simulink model "MODEL_PV"  (R2024a)
settings: Solver=VariableStepAuto  StartTime=0.0  StopTime=120  RelTol=1e-3
PostLoadFcn:
  | setup_01
model workspace (MAT data in the model file):
  TrafficLightPosition = [-6.9 -1.9 8]
  egoVelocity = 9
  relDist = inf
  relVelMIO = inf
  timeGap = 0.9
  trafficLightSensorStates = 1
undefined symbols (not defined in the file): costmap, intersectionInfo, maxMIOLeadDistance, posSelector, referencePathInfo, routePlan, sceneOrigin, Ts, v_set, velSelector
libraries: drivingscenarioandsensors x2, drivingvehiclecontroller x1
CloseFcn:
  | clearvars -except out
settings Model: PacingRate=0.500000  Creator=fidel  LastModifiedBy=L03509110
settings OptimizationCC: ReuseModelBlockBuffer=off
settings RTWCC: GPUComputeCapability=3.5

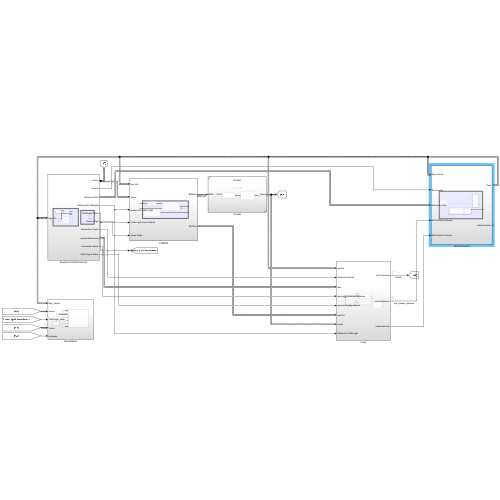
[thumbnail: Simulink's stored preview of the top-level diagram]
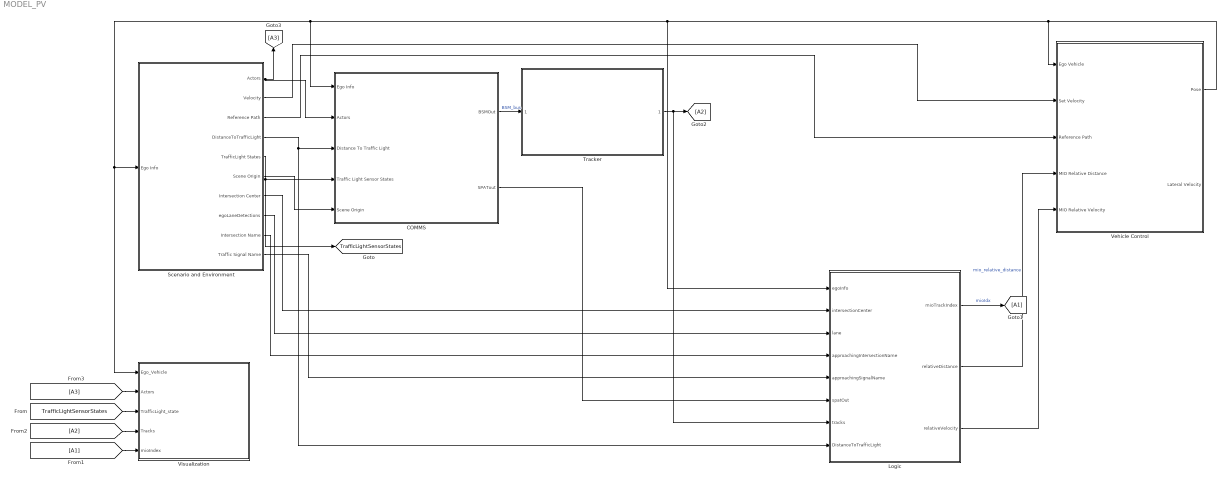
== system MODEL_PV ==
  COMMS : Subsystem
  Logic : Subsystem
  Scenario and Environment : Subsystem
  Tracker : Subsystem  ReferencedSubsystem=Tracker
  Vehicle Control : Subsystem
  Visualization : Subsystem
  tag scope: TrafficLightSensorStates=global
  wires:
  Vehicle Control/1(Pose) -> Vehicle Control/1(Ego Vehicle), Logic/1(egoInfo), COMMS/1(Ego Info), Visualization/1(Ego_Vehicle), Scenario and Environment/1(Ego Info)
  Scenario and Environment/3(Reference Path) -> Vehicle Control/3(Reference Path)
  [A3] -> Visualization/2(Actors)
  Scenario and Environment/1(Actors) -> [A3], COMMS/2(Actors)
  [TrafficLightSensorStates] -> Visualization/3(TrafficLight_state)
  [A2] -> Visualization/4(Tracks)
  [A1] -> Visualization/5(mioIndex)
  Scenario and Environment/2(Velocity) -> Vehicle Control/2(Set Velocity)
  Scenario and Environment/4(DistanceToTrafficLight) -> Logic/8(DistanceToTrafficLight), COMMS/3("Distance To Traffic Light ")
  Scenario and Environment/5(TrafficLight States) -> [TrafficLightSensorStates], COMMS/4(Traffic Light Sensor States)
  Scenario and Environment/6(Scene Origin) -> COMMS/5(Scene Origin)
  COMMS/1(BSMOut) -> Tracker/1  "BSM_bus"
  Scenario and Environment/7(Intersection Center) -> Logic/2(intersectionCenter)
  Scenario and Environment/8(egoLaneDetections) -> Logic/3(lane)
  Scenario and Environment/9(Intersection Name) -> Logic/4(approachingIntersectionName)
  Scenario and Environment/10(Traffic Signal Name) -> Logic/5(approachingSignalName)
  Logic/1(mioTrackIndex) -> [A1]  "mioIdx"
  COMMS/2(SPATout) -> Logic/6(spatOut)
  Tracker/1 -> [A2], Logic/7(tracks)
  Logic/2(relativeDistance) -> Vehicle Control/4(MIO Relative Distance)  "mio_relative_distance"
  Logic/3(relativeVelocity) -> Vehicle Control/5(MIO Relative Velocity)

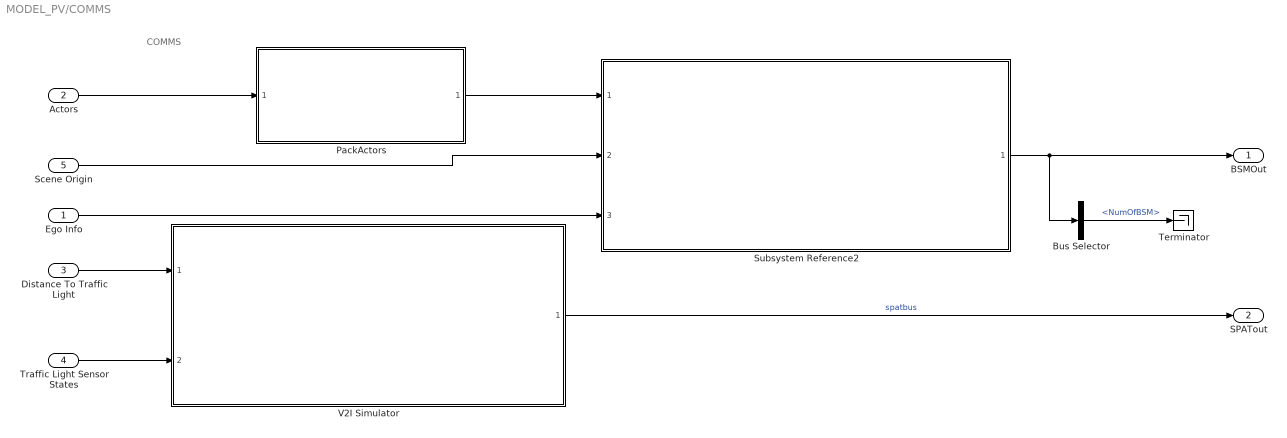
== system MODEL_PV/COMMS ==
  note: COMMS
  Ego Info : Inport
  Actors : Inport  Port=2
  "Distance To Traffic Light " : Inport  Port=3
  Traffic Light Sensor States : Inport  Port=4
  Scene Origin : Inport  Port=5
  Bus Selector : BusSelector  OutputSignals=NumOfBSM
  PackActors : Subsystem  ReferencedSubsystem=Pack_Actors_Info
  Subsystem Reference2 : Subsystem  ReferencedSubsystem=V2VSimulator
  Terminator : Terminator
  V2I Simulator : Subsystem  ReferencedSubsystem=V2ISimulator
  BSMOut : Outport
  SPATout : Outport  Port=2
  wires:
  PackActors/1 -> Subsystem Reference2/1
  Ego Info/1 -> Subsystem Reference2/3
  Scene Origin/1 -> Subsystem Reference2/2
  Traffic Light Sensor States/1 -> V2I Simulator/2
  Subsystem Reference2/1 -> Bus Selector/1, BSMOut/1
  V2I Simulator/1 -> SPATout/1  "spatbus"
  Actors/1 -> PackActors/1
  "Distance To Traffic Light "/1 -> V2I Simulator/1
  Bus Selector/1 -> Terminator/1  "<NumOfBSM>"

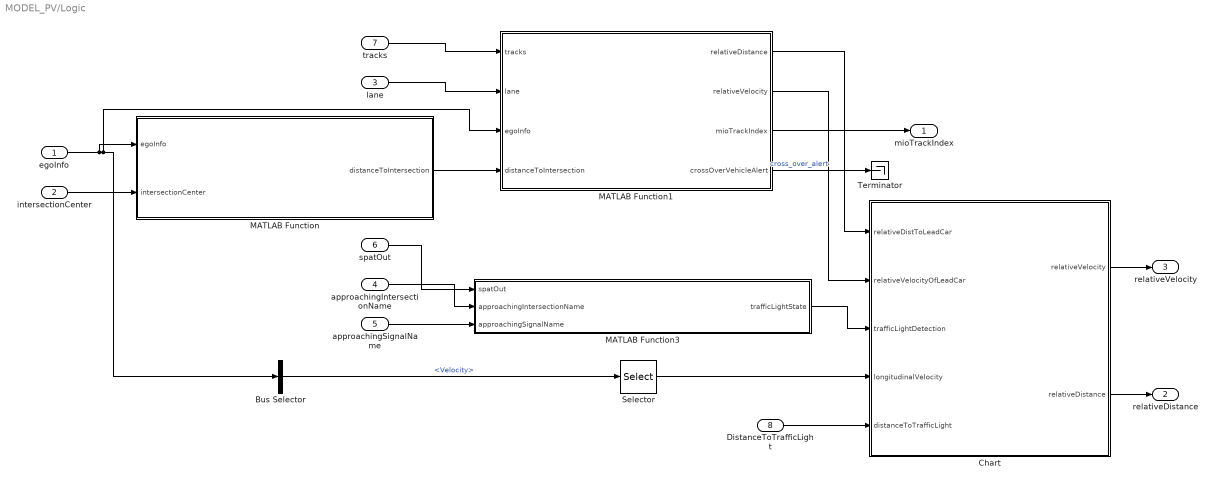
== system MODEL_PV/Logic ==
  egoInfo : Inport
  intersectionCenter : Inport  Port=2
  lane : Inport  Port=3
  approachingIntersectionName : Inport  Port=4
  approachingSignalName : Inport  Port=5
  spatOut : Inport  Port=6
  tracks : Inport  Port=7
  DistanceToTrafficLight : Inport  Port=8
  Bus Selector : BusSelector  OutputSignals=Velocity
  Chart : Stateflow chart  TreatAsAtomicUnit=on
  MATLAB Function : MATLAB Function  TreatAsAtomicUnit=on
  MATLAB Function1 : MATLAB Function  TreatAsAtomicUnit=on  mask{maxDistance=maxMIOLeadDistance, posSelector=posSelector, velSelector=velSelector}
      mask prompts: maxDistance "Maximum lead distance"; posSelector "Track Position Selector"; velSelector "Track Velocity Selector"
  MATLAB Function3 : MATLAB Function  TreatAsAtomicUnit=on
  Selector : Selector  InputPortWidth=3  IndexOptions=Index vector (dialog)  Indices=[1]  OutputSizes=1
  Terminator : Terminator
  mioTrackIndex : Outport
  relativeDistance : Outport  Port=2
  relativeVelocity : Outport  Port=3
  wires:
  egoInfo/1 -> MATLAB Function1/3(egoInfo), Bus Selector/1, MATLAB Function/1(egoInfo)
  intersectionCenter/1 -> MATLAB Function/2(intersectionCenter)
  Chart/1(relativeVelocity) -> relativeVelocity/1
  tracks/1 -> MATLAB Function1/1(tracks)
  lane/1 -> MATLAB Function1/2(lane)
  spatOut/1 -> MATLAB Function3/1(spatOut)
  approachingIntersectionName/1 -> MATLAB Function3/2(approachingIntersectionName)
  approachingSignalName/1 -> MATLAB Function3/3(approachingSignalName)
  MATLAB Function/1(distanceToIntersection) -> MATLAB Function1/4(distanceToIntersection)
  Chart/2(relativeDistance) -> relativeDistance/1
  Bus Selector/1 -> Selector/1  "<Velocity>"
  MATLAB Function1/1(relativeDistance) -> Chart/1(relativeDistToLeadCar)
  MATLAB Function1/2(relativeVelocity) -> Chart/2(relativeVelocityOfLeadCar)
  MATLAB Function1/3(mioTrackIndex) -> mioTrackIndex/1
  MATLAB Function3/1(trafficLightState) -> Chart/3(trafficLightDetection)
  Selector/1 -> Chart/4(longitudinalVelocity)
  DistanceToTrafficLight/1 -> Chart/5(distanceToTrafficLight)
  MATLAB Function1/4(crossOverVehicleAlert) -> Terminator/1  "cross_over_alert"

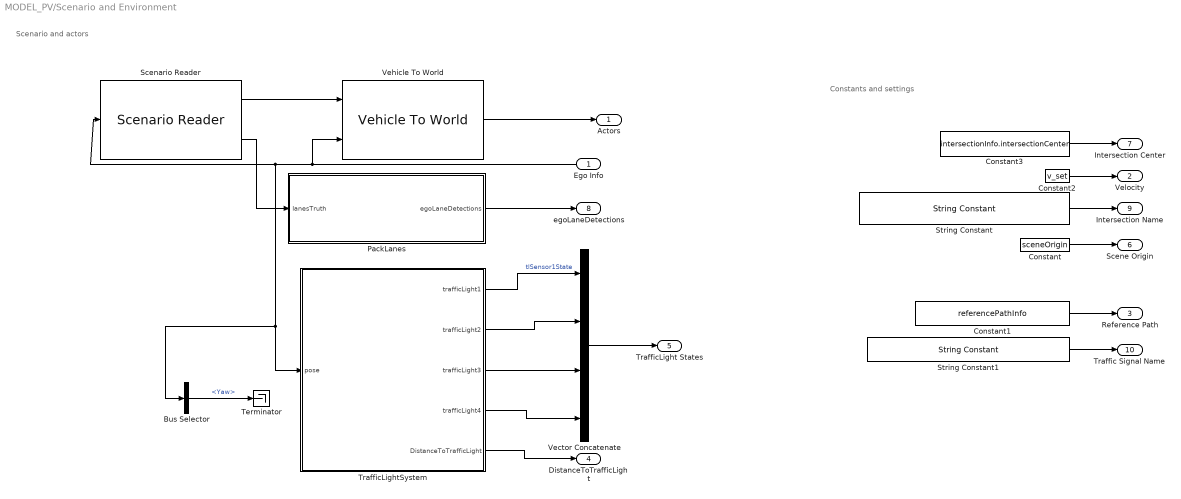
== system MODEL_PV/Scenario and Environment ==
  note: Scenario and actors
  note: Constants and settings
  Ego Info : Inport
  Bus Selector : BusSelector  OutputSignals=Yaw
  Constant : Constant  Value=sceneOrigin
  Constant1 : Constant  Value=referencePathInfo  OutDataTypeStr=Bus: ReferencePathInfo  SampleTime=0.1  LockScale=on
  Constant2 : Constant  Value=v_set  SampleTime=Ts
  Constant3 : Constant  Value=intersectionInfo.intersectionCenter  SampleTime=Ts
  PackLanes : MATLAB Function  TreatAsAtomicUnit=on  mask{detStructObj=Simulink.Bus.createMATLABStruct('LaneSensor')}
      mask prompts: detStructObj "Output lane detections struct"
  Scenario Reader : drivingscenarioandsensors/Scenario Reader  ScenarioSource=From workspace  ScenarioFileName=EgoVehicleGoesStraight.mat  ScenarioVariableName=scenario  OutputCoordinateSystem=Vehicle coordinates  EgoVehicleSource=Input port  EgoVehicleActorID=egoVehicle.ActorID  OrientVehiclesOnRoad=off  OutputEgoVehiclePose=on  OutputEgoVehicleState=off  SampleTime=0.1  LaneBoundaryOutput=Ego vehicle lane boundaries  LaneBoundaryDistance=0:0.5:9.5  LaneBoundaryLocation=Center of lane markings  BusNameSource=Property  BusName=BusActors  BusNumActorsSource=Property  BusNumActors=12  BusName2Source=Property  BusName2=BusLaneBoundaries  BusNumLaneBoundariesSource=Scenario  BusNumLaneBoundaries=10  BusName3Source=Auto  BusName3=BusEgoActor  BusName4Source=Auto  BusName4=BusEgoState  ShowCoordinateLabels=on  SimulateUsing=Interpreted execution
  String Constant : StringConstant  String=approachingIntersectionName
  String Constant1 : StringConstant  String=approachingSignalName
  Terminator : Terminator
  TrafficLightSystem : Subsystem  mask{TrafficLightSensorModeSelection=Cycle}
  Vector Concatenate : Concatenate  NumInputs=4  Mode=Multidimensional array
  Vehicle To World : drivingscenarioandsensors/Vehicle To World  BusNameSource=Property  BusName=BusVehicleToWorldActors  SimulateUsing=Interpreted execution
  Actors : Outport
  Velocity : Outport  Port=2
  Reference Path : Outport  Port=3
  DistanceToTrafficLight : Outport  Port=4
  TrafficLight States : Outport  Port=5
  Scene Origin : Outport  Port=6
  Intersection Center : Outport  Port=7
  egoLaneDetections : Outport  Port=8
  Intersection Name : Outport  Port=9
  Traffic Signal Name : Outport  Port=10
  wires:
  Constant/1 -> Scene Origin/1
  Constant2/1 -> Velocity/1
  Constant1/1 -> Reference Path/1
  Constant3/1 -> Intersection Center/1
  String Constant/1 -> Intersection Name/1
  String Constant1/1 -> Traffic Signal Name/1
  Scenario Reader/2 -> PackLanes/1(lanesTruth)
  Scenario Reader/1 -> Vehicle To World/1
  Vehicle To World/1 -> Actors/1
  PackLanes/1(egoLaneDetections) -> egoLaneDetections/1
  TrafficLightSystem/1(trafficLight1) -> Vector Concatenate/1  "tlSensor1State"
  Ego Info/1 -> Scenario Reader/1, Bus Selector/1, TrafficLightSystem/1(pose), Vehicle To World/2
  TrafficLightSystem/2(trafficLight2) -> Vector Concatenate/2
  TrafficLightSystem/3(trafficLight3) -> Vector Concatenate/3
  TrafficLightSystem/4(trafficLight4) -> Vector Concatenate/4
  TrafficLightSystem/5(DistanceToTrafficLight) -> DistanceToTrafficLight/1
  Vector Concatenate/1 -> TrafficLight States/1
  Bus Selector/1 -> Terminator/1  "<Yaw>"

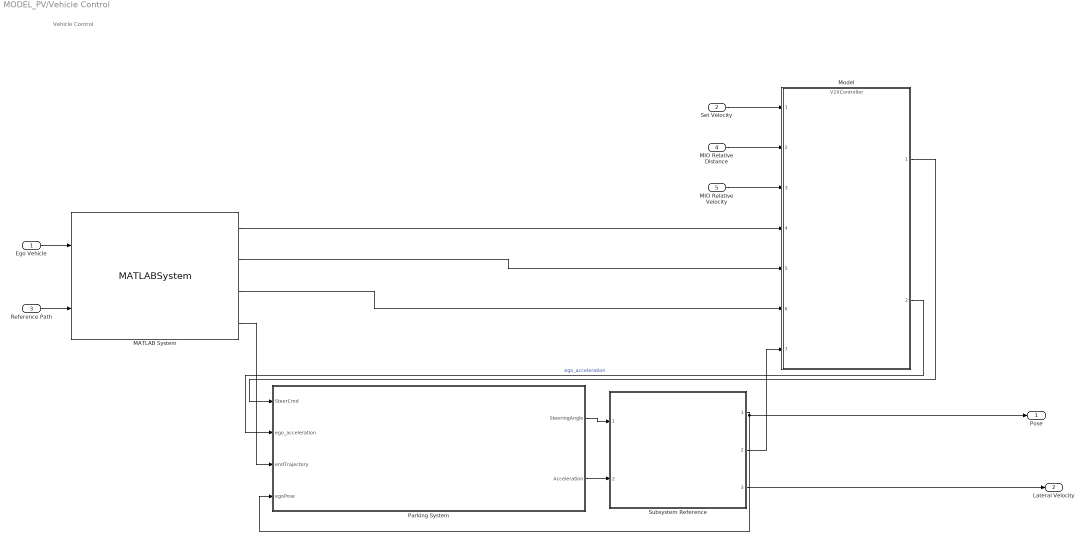
== system MODEL_PV/Vehicle Control ==
  note: Vehicle Control
  Ego Vehicle : Inport
  Set Velocity : Inport  Port=2
  Reference Path : Inport  Port=3
  MIO Relative Distance : Inport  Port=4  SampleTime=Ts
  MIO Relative Velocity : Inport  Port=5  SampleTime=Ts
  MATLAB System : MATLABSystem  System=CalculateReferencePose  PredictionHorizon=PredictionHorizon  DistanceFromCGToRear=lr  SampleTime=0.1  SimulateUsing=Code generation
      mask Type: CalculateReferencePose
      mask Display:
      | disp('CalculateReferencePose');
      | port_label('input',1,'EgoActor');
      | port_label('input',2,'EgoReferencePath');
      | port_label('output',1,'CurvatureSequence');
      | port_label('output',2,'LateralDeviation');
      | port_label('output',3,'RelativeYawAngle');
      | port_label('output',4,'IsGoalReached');
  Model : ModelReference  ModelNameDialog=V2XController.slx  SimulationMode=Normal  ModelReferenceVersion=4.1
  Parking System : Subsystem
  Subsystem Reference : Subsystem  ReferencedSubsystem=VehicleDynamics
  Pose : Outport
  Lateral Velocity : Outport  Port=2
  wires:
  Reference Path/1 -> MATLAB System/2
  MIO Relative Velocity/1 -> Model/3
  Ego Vehicle/1 -> MATLAB System/1
  MATLAB System/1 -> Model/4
  Parking System/1(SteeringAngle) -> Subsystem Reference/1
  MATLAB System/2 -> Model/5
  Parking System/2(Acceleration) -> Subsystem Reference/2
  MATLAB System/3 -> Model/6
  MATLAB System/4 -> Parking System/3(endTrajectory)
  Set Velocity/1 -> Model/1
  MIO Relative Distance/1 -> Model/2
  Subsystem Reference/1 -> Parking System/4(egoPose), Pose/1
  Subsystem Reference/2 -> Model/7
  Subsystem Reference/3 -> Lateral Velocity/1
  Model/1 -> Parking System/1(SteerCmd)
  Model/2 -> Parking System/2(ego_acceleration)  "ego_acceleration"

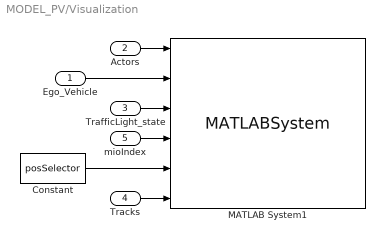
== system MODEL_PV/Visualization ==
  Ego_Vehicle : Inport
  Actors : Inport  Port=2
  TrafficLight_state : Inport  Port=3
  Tracks : Inport  Port=4
  mioIndex : Inport  Port=5
  Constant : Constant  Value=posSelector
  MATLAB System1 : MATLABSystem  System=visualizationS2  range=V2XRange  SF_std=SF_std  TrafficLightDisp=on  EnableVisualization=on
      mask Type: visualizationS2
      mask Display:
      | disp('visualizationS2');
      | port_label('input',1,'targetPoses');
      | port_label('input',2,'egoInfo');
      | port_label('input',3,'trafficLightSensorStates');
      | port_label('input',4,'mioIndex');
      | port_label('input',5,'posSelector');
      | port_label('input',6,'tracks');
  wires:
  TrafficLight_state/1 -> MATLAB System1/3
  Actors/1 -> MATLAB System1/1
  Ego_Vehicle/1 -> MATLAB System1/2
  Tracks/1 -> MATLAB System1/6
  mioIndex/1 -> MATLAB System1/4
  Constant/1 -> MATLAB System1/5

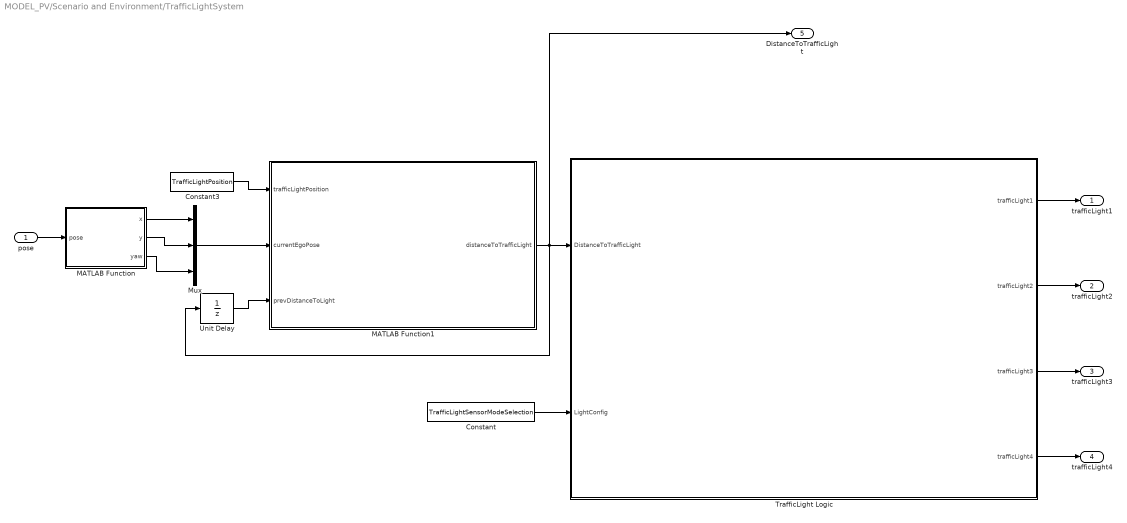
== system MODEL_PV/Scenario and Environment/TrafficLightSystem ==
  pose : Inport
  Constant : Constant  Value=TrafficLightSensorModeSelection
  Constant3 : Constant  Value=TrafficLightPosition
  MATLAB Function : MATLAB Function  TreatAsAtomicUnit=on
  MATLAB Function1 : MATLAB Function  TreatAsAtomicUnit=on  mask{minTLDist=3}
      mask prompts: minTLDist "Minimum distance to traffic light"
  Mux : Mux  Inputs=3
  TrafficLight Logic : Stateflow chart  TreatAsAtomicUnit=on
  Unit Delay : UnitDelay  InitialCondition=100  SampleTime=-1  HasFrameUpgradeWarning=on
  trafficLight1 : Outport
  trafficLight2 : Outport  Port=2
  trafficLight3 : Outport  Port=3
  trafficLight4 : Outport  Port=4
  DistanceToTrafficLight : Outport  Port=5
  wires:
  pose/1 -> MATLAB Function/1(pose)
  Mux/1 -> MATLAB Function1/2(currentEgoPose)
  Unit Delay/1 -> MATLAB Function1/3(prevDistanceToLight)
  Constant3/1 -> MATLAB Function1/1(trafficLightPosition)
  MATLAB Function/3(yaw) -> Mux/3
  MATLAB Function/2(y) -> Mux/2
  MATLAB Function/1(x) -> Mux/1
  MATLAB Function1/1(distanceToTrafficLight) -> DistanceToTrafficLight/1, Unit Delay/1, TrafficLight Logic/1(DistanceToTrafficLight)
  Constant/1 -> TrafficLight Logic/2(LightConfig)
  TrafficLight Logic/1(trafficLight1) -> trafficLight1/1
  TrafficLight Logic/2(trafficLight2) -> trafficLight2/1
  TrafficLight Logic/3(trafficLight3) -> trafficLight3/1
  TrafficLight Logic/4(trafficLight4) -> trafficLight4/1

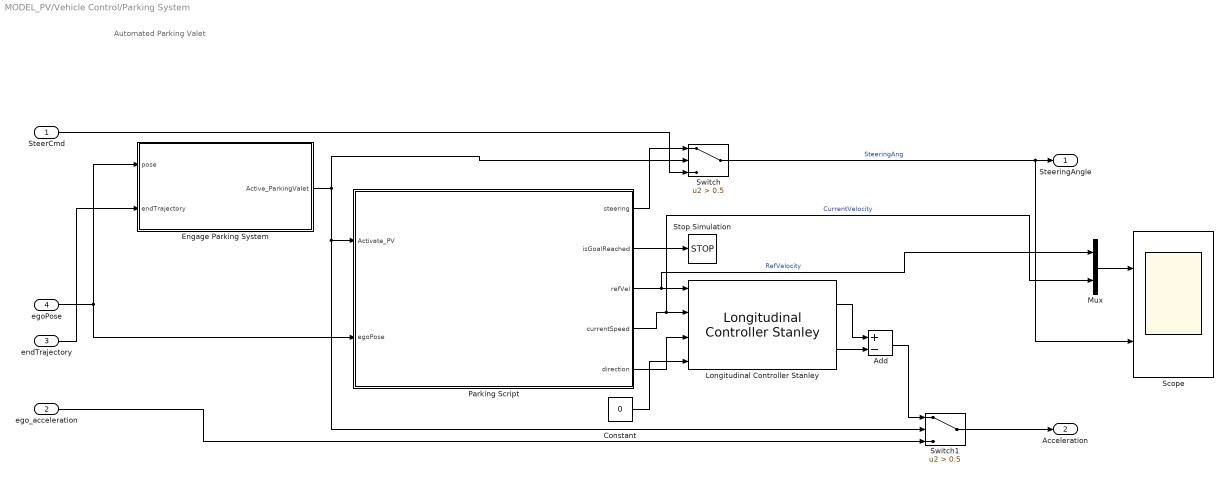
== system MODEL_PV/Vehicle Control/Parking System ==
  note: Automated Parking Valet
  SteerCmd : Inport
  ego_acceleration : Inport  Port=2
  endTrajectory : Inport  Port=3
  egoPose : Inport  Port=4
  Add : Sum  Inputs=+-
  Constant : Constant  Value=0
  Engage Parking System : MATLAB Function  TreatAsAtomicUnit=on
  Longitudinal Controller Stanley : drivingvehiclecontroller/Longitudinal Controller Stanley  Kp=2.5  Ki=1  SampleTime=0.05  MaxAcceleration=3  MaxDeceleration=6
  Mux : Mux  Inputs=2
  Parking Script : MATLAB Function  TreatAsAtomicUnit=on  mask{Costmap=costmap, RoutePlan=routePlan}
      mask init:
      | validateattributes(Costmap, {'vehicleCostmap'}, {'scalar'});
      | validateattributes(RoutePlan, {'table'}, {'ncols', 3});
      | 
      | routePlanStruct   = table2struct(RoutePlan);
      | varagout          = helperSLCreateUtilityStruct(Costmap);
      | vehicleDimsStruct = varagout{1};
      | costmapStruct     = varagout{2};
  Scope : Scope  NumInputPorts=2
  Stop Simulation : Stop
  Switch : Switch  Criteria=u2 > Threshold  Threshold=0.5  SaturateOnIntegerOverflow=off  InputSameDT=off
  Switch1 : Switch  Criteria=u2 > Threshold  Threshold=0.5  SaturateOnIntegerOverflow=off  InputSameDT=off
  SteeringAngle : Outport
  Acceleration : Outport  Port=2
  wires:
  Constant/1 -> Longitudinal Controller Stanley/4
  Engage Parking System/1(Active_ParkingValet) -> Switch/2, Switch1/2, Parking Script/1(Activate_PV)
  SteerCmd/1 -> Switch/3
  Parking Script/5(direction) -> Longitudinal Controller Stanley/3
  Parking Script/4(currentSpeed) -> Mux/2, Longitudinal Controller Stanley/2  "CurrentVelocity"
  Parking Script/3(refVel) -> Mux/1, Longitudinal Controller Stanley/1  "RefVelocity"
  Parking Script/2(isGoalReached) -> Stop Simulation/1
  Parking Script/1(steering) -> Switch/1
  Add/1 -> Switch1/1
  Longitudinal Controller Stanley/1 -> Add/1
  Longitudinal Controller Stanley/2 -> Add/2
  egoPose/1 -> Engage Parking System/1(pose), Parking Script/2(egoPose)
  Switch/1 -> SteeringAngle/1, Scope/2  "SteeringAng"
  Switch1/1 -> Acceleration/1
  endTrajectory/1 -> Engage Parking System/2(endTrajectory)
  ego_acceleration/1 -> Switch1/3
  Mux/1 -> Scope/1

== matlab function MODEL_PV/Scenario and Environment/PackLanes ==
  data: lanesTruth input; egoLaneDetections output Bus: LaneSensor; detStructObj parameter
function egoLaneDetections = packLanesTruth(lanesTruth, detStructObj)
% Assign lane parameters from ground-truth lane boundaries.

% Assign lane detections struct object to output variable
egoLaneDetections = detStructObj;

% Find ego-vehicle lane boundary indices
lbNum = [1, 1];
for j = 1:length(lanesTruth.LaneBoundaries)-1
    yleftLane = lanesTruth.LaneBoundaries(j+1).Coordinates(1,2);
    yrightLane = lanesTruth.LaneBoundaries(j).Coordinates(1,2);
    
    if ((0 >= yleftLane) && (0 <= yrightLane))
        lbNum(1) = j;
        lbNum(2) = j+1;
        break;
    elseif ((0 >= yrightLane) && (0 <= yleftLane))
        lbNum(1) = j+1;
        lbNum(2) = j;
        break;
    end
end

%% Pack left lane info
coder.varsize('leftLaneCoordinates')
leftLaneCoordinates = lanesTruth.LaneBoundaries(lbNum(1)).Coordinates;
idx = ~isfinite(leftLaneCoordinates(:,1));
leftLaneCoordinates(idx,:) = [];
if size(leftLaneCoordinates,1) > 2
    % Get parabolic lane boundary parameters using polyfit for the left lane.
    leftLaneParameters = polyfit(leftLaneCoordinates(:,1),...
        leftLaneCoordinates(:,2),2);
    
    % Assign left lane parameters to output bus, lanes.
    egoLaneDetections.Left.Curvature = single(2 * leftLaneParameters(1));
    egoLaneDetections.Left.HeadingAngle = single(leftLaneParameters(2));
    egoLaneDetections.Left.LateralOffset = single(leftLaneParameters(3));
    
    egoLaneDetections.Left.Strength = single(lanesTruth.LaneBoundaries(lbNum(1)).Strength);
end


%% Pack right lane info
coder.varsize('rightLaneCoordinates')
rightLaneCoordinates = lanesTruth.LaneBoundaries(lbNum(2)).Coordinates;
idx = ~isfinite(rightLaneCoordinates(:,1));
rightLaneCoordinates(idx,:) = [];
if size(rightLaneCoordinates,1) > 2
    % Get parabolic lane boundary parameters using polyfit for the right lane
    rightLaneParameters = polyfit(rightLaneCoordinates(:,1),...
        rightLaneCoordinates(:,2),2);
    
    % Assign right lane parameters to output bus, lanes.
    egoLaneDetections.Right.Curvature = single(2 * rightLaneParameters(1));
    egoLaneDetections.Right.HeadingAngle = single(rightLaneParameters(2));
    egoLaneDetections.Right.LateralOffset = single(rightLaneParameters(3));
    
    egoLaneDetections.Right.Strength = single(lanesTruth.LaneBoundaries(lbNum(2)).Strength);
end
end

== stateflow chart MODEL_PV/Logic/Chart ==
  state OnEntry
    entry:
    relativeDistance = relativeDistToLeadCar;
    relativeVelocity = relativeVelocityOfLeadCar;
  state OnRedAndYellowLightDetection
    entry:
    relativeDistance = min(relativeDistToLeadCar,distanceToTrafficLight);
    relativeVelocity = min(relativeVelocityOfLeadCar,longitudinalVelocity);
  (default) -> OnEntry
  OnEntry -> OnEntry [order 2] : [hasChanged(relativeDistToLeadCar)]
  OnRedAndYellowLightDetection -> OnEntry [order 1] : [trafficLightDetection==Green || trafficLightDetection == NoDetections ]
  OnEntry -> OnRedAndYellowLightDetection [order 1] : [(trafficLightDetection==Red || trafficLightDetection==Yellow) && distanceToTrafficLight ~= inf]
  OnRedAndYellowLightDetection -> OnRedAndYellowLightDetection [order 2] : [hasChanged(relativeDistToLeadCar)]
  OnRedAndYellowLightDetection -> OnRedAndYellowLightDetection [order 3] : [hasChanged(distanceToTrafficLight)]
  data: Green local =2; Red local =0; Yellow local =1; NoDetections local =-1; relativeVelocity output; relativeDistance output; relativeDistToLeadCar input; relativeVelocityOfLeadCar input; trafficLightDetection input; longitudinalVelocity input; distanceToTrafficLight input

== matlab function MODEL_PV/Logic/MATLAB Function3 ==
  data: spatOut input; trafficLightState output; approachingIntersectionName input; approachingSignalName input
function trafficLightState = extractTrafficLightDetection(spatOut,approachingIntersectionName,approachingSignalName)
%     approachingIntersectionName = "TrafficLightGroup_1";
%     approachingSignalName = "TrafficLight_1";
    trafficLightState = -1;
    coder.extrinsic("GetTrafficLightDetection")
    trafficLightState = GetTrafficLightDetection(spatOut,approachingIntersectionName,approachingSignalName);
end

== matlab function MODEL_PV/Vehicle Control/Parking System/Parking Script ==
  data: Activate_PV input; egoPose input; steering output; isGoalReached output; refVel output; currentSpeed output; direction output; vehicleDimsStruct parameter; routePlanStruct parameter; costmapStruct parameter
function [steering, isGoalReached, refVel, currentSpeed, direction] = fcn(Activate_PV, egoPose, vehicleDimsStruct, routePlanStruct, costmapStruct)

%#codegen

% Salida default hasta que no se active el modo parking
isGoalReached = false;
steering=0;
refVel=0;
currentSpeed=0;
direction=1;
%

% Variables para el sistema, determinadas desde la simulación 2D
maxLocalPlanDistance = 2; % in meters
minTurningRadius=5;
RRTConnectionDistance=3;
ConstantVel=2;   
%

% persistent variables para que se mantengan de una ejecución a la otra
persistent behavioralPlanner pathAnalyzer 
persistent plannerConfig costmap motionPlanner
persistent nextGoalPose refPath directionsInternal posesInternal nextGoal


if Activate_PV==1

    currentPose = [egoPose.Position(2)+8 egoPose.Position(1)-8 egoPose.Yaw+90].*[-1 1 1];
    currentSpeed= norm(egoPose.Velocity);
    
    

    if isempty(behavioralPlanner)
    % Initialize Route planner
    steerLimit = 30;
    behavioralPlanner = HelperBehavioralPlanner(routePlanStruct, steerLimit);
    
    % [nextGoal, plannerConfig, speedConfig] = requestManeuver( ...
    %     behavioralPlanner, currentPose, currentSpeed);

    % HelperPathAnalyzer>| object to compute reference pose, reference velocity
    % and driving direction for the controller.
    pathAnalyzer = HelperPathAnalyzer(Wheelbase=vehicleDimsStruct.Wheelbase);

    weights = struct(Time=10, Smoothness=100, Obstacle=50);
    vehicleInfo = struct("Dimension", [vehicleDimsStruct.Length, vehicleDimsStruct.Width], "Shape", "Rectangle");

    % Create vehicleDimensions object
    vehicleDims = vehicleDimensions( ...
    vehicleDimsStruct.Length, ...
    vehicleDimsStruct.Width, ...
    vehicleDimsStruct.Height, ...
    'Wheelbase',          vehicleDimsStruct.Wheelbase, ...
    'RearOverhang',       vehicleDimsStruct.RearOverhang, ...
    'WorldUnits',         char(vehicleDimsStruct.WorldUnits));
       

    ccConfig = inflationCollisionChecker(vehicleDims, 4);

    % Initialize vehicleCostmap object
    costmap = vehicleCostmap(costmapStruct.Costs, ...
        'FreeThreshold',      costmapStruct.FreeThreshold, ...
        'OccupiedThreshold',  costmapStruct.OccupiedThreshold, ...
        'MapLocation',        costmapStruct.MapExtent([1, 3]), ...
        'CellSize',           costmapStruct.CellSize, ...
        'CollisionChecker',   ccConfig);

    %Create pathPlannerRRT object
    motionPlanner = pathPlannerRRT(costmap, ...
        'ConnectionDistance', RRTConnectionDistance, ...
        'MinIterations',      1000, ...
        'GoalTolerance',      [0.5	0.5	10], ...
        'MinTurningRadius',   minTurningRadius);

    end
    
    % Initialize persistent variables
    if isempty(nextGoalPose)
        nextGoalPose = [0 0 0];
    end
    
    if isempty(posesInternal)
        posesInternal = [0 0 0];
    end
    
    if isempty(directionsInternal)
        directionsInternal = 1;
    end

    if isempty(nextGoal)
        nextGoal = [0 0 0];
    end
    

  
    if planNextSegment(behavioralPlanner, currentPose, 2*maxLocalPlanDistance)
        [nextGoal, plannerConfig, speedConfig] = requestManeuver( ...
        behavioralPlanner, currentPose, currentSpeed);
        nextGoalPose  = nextGoal;
        vehiclePose   = currentPose;
        refPath       = plan(motionPlanner, vehiclePose, nextGoalPose);
        [refPoses, directions] = interpolate(refPath);
        posesInternal          = refPoses;
        directionsInternal     = directions;
    end

    refPoses   = posesInternal;
    directions = directionsInternal;
    


    % Configure path analyzer.
    pathAnalyzer.RefPoses     = refPoses;
    pathAnalyzer.Directions   = directions;
    pathAnalyzer.VelocityProfile = ConstantVel*ones(length(directions),1);

    % Find the reference pose on the path and the corresponding
    % velocity.
    [refPose, refVel, direction] = pathAnalyzer(currentPose, currentSpeed);

    % Compute steering command.
    steeringAngle = lateralControllerStanley(refPose, currentPose, currentSpeed, ...
        Direction=direction, Wheelbase=vehicleDimsStruct.Wheelbase, PositionGain=4);


    steering=deg2rad(-steeringAngle);


    isGoalReached=helperGoalChecker(nextGoal, currentPose, currentSpeed, ConstantVel, direction);

end

== matlab function MODEL_PV/Scenario and Environment/TrafficLightSystem/MATLAB Function1 ==
  data: trafficLightPosition input; distanceToTrafficLight output; currentEgoPose input; minTLDist parameter; prevDistanceToLight input
function distanceToTrafficLight   = computeDistanceToTrafficLight(trafficLightPosition, currentEgoPose, minTLDist, prevDistanceToLight)
    % helperComputeDistanceToTrafficLight Compute distance to upcoming traffic
    % light.
    %
    % Current Ego position and the upcoming traffic light position information
    % are used for calculating distance to traffic light. 
    %
    % NOTE: This is a helper function for example purposes and may be removed or
    % modified in the future.
    %
    
    % Copyright 2021 The MathWorks, Inc.
    
    % Once the vehicle reaches the traffic light, it should see the next
    % traffic light if any. In this example, there is no next traffic light so
    % the next traffic light is assumed at infinite distance. 
    %
    % if the previous distance between the vehicle and the traffic light is
    % less than the minTLDist, then it is treated that vehicle has passed the
    % light.
    
    if(prevDistanceToLight < minTLDist || prevDistanceToLight == Inf)
        distanceToTrafficLight = inf;
    else
        % Euclidean distance to upcoming traffic light from the current
        % position of ego vehicle.
        %
        distanceToTrafficLight = double(sqrt((trafficLightPosition(1)-currentEgoPose(1))^2 + ...
            (trafficLightPosition(2)-currentEgoPose(2))^2));
    end
end

== matlab function MODEL_PV/Scenario and Environment/TrafficLightSystem/MATLAB Function ==
  data: x output; pose input; y output; yaw output
function [x, y, yaw] = poseToSim(pose)

pos_Rr = pose.Position([1,2])';
theta = pose.Yaw;

pos_Cen = pos_Rr+[cosd(theta) sind(theta)]';

x = pos_Cen(1);
y = pos_Cen(2);
yaw = pose.Yaw;

== stateflow chart MODEL_PV/Scenario and Environment/TrafficLightSystem/TrafficLight Logic ==
  state STEADYGREEN
    entry:
    trafficLight1 = Green;
    trafficLight2 = Red;
    trafficLight3 = Green;
    trafficLight4 = Red;
  state START
    entry:
    trafficLight1 = Red;
    trafficLight2 = Red;
    trafficLight3 = Red;
    trafficLight4 = Red;
  state STEADYRED
    entry:
    trafficLight1 = Red;
    trafficLight2 = Green;
    trafficLight3 = Red;
    trafficLight4 = Green;
  state TRAFFICLIGHT1YELLOW
    entry:
    trafficLight1 = Yellow;
    trafficLight2 = Red;
    trafficLight3 = Yellow;
    trafficLight4 = Red;
  state TRAFFICLIGHT1GREEN
    entry:
    trafficLight1 = Green;
    trafficLight2 = Red;
    trafficLight3 = Green;
    trafficLight4 = Red;
  state TRAFFICLIGHT2GREEN
    entry:
    trafficLight1 = Red;
    trafficLight2 = Green;
    trafficLight3 = Red;
    trafficLight4 = Green;
  state TRAFFICLIGHT2YELLOW
    entry:
    trafficLight1 = Red;
    trafficLight2 = Yellow;
    trafficLight3 = Red;
    trafficLight4 = Yellow;
  (default) -> START
  START -> STEADYGREEN [order 1] : [DistanceToTrafficLight < trafficLightStateTriggerThreshold ...
      |  && LightConfig==1]
  START -> STEADYRED [order 3] : [DistanceToTrafficLight < trafficLightStateTriggerThreshold ...
      | && LightConfig==2]
  START -> TRAFFICLIGHT1GREEN [order 2] : [DistanceToTrafficLight < trafficLightStateTriggerThreshold && LightConfig ==3]
  TRAFFICLIGHT1GREEN -> TRAFFICLIGHT1YELLOW : after(4.2, sec)
  TRAFFICLIGHT1YELLOW -> TRAFFICLIGHT2GREEN : after(0.5,sec)
  TRAFFICLIGHT2YELLOW -> TRAFFICLIGHT1GREEN : after(0.5,sec)
  TRAFFICLIGHT2GREEN -> TRAFFICLIGHT2YELLOW : after(4,sec)
  data: DistanceToTrafficLight input; Green constant double =2; Red constant double =0; LightConfig input; trafficLightStateTriggerThreshold parameter; trafficLight1 output; trafficLight2 output; trafficLight3 output; trafficLight4 output; Yellow constant double =1

== matlab function MODEL_PV/Vehicle Control/Parking System/Engage Parking System ==
  settings: sampleTime=Ts
  data: pose input; Active_ParkingValet output; endTrajectory input
function Active_ParkingValet = fcn(pose, endTrajectory)

Active_ParkingValet=0;


if endTrajectory

    
    currentEgoPose = pose.Position;

    if (currentEgoPose(1)>8) && (currentEgoPose(1)<59) && (currentEgoPose(2)>-59) && (currentEgoPose(2)<-8)

        Active_ParkingValet=1;
    end


end

== matlab function MODEL_PV/Logic/MATLAB Function ==
  data: egoInfo input; distanceToIntersection output; intersectionCenter input
function distanceToIntersection = computeDistanceToIntersection(egoInfo,intersectionCenter)

currentEgoPose = [0 0 0];
currentEgoPose = egoInfo.Position;
distanceToIntersection = double(sqrt((intersectionCenter(1)- ...
    currentEgoPose(1))^2 + (intersectionCenter(2)- currentEgoPose(2))^2));

end

== matlab function MODEL_PV/Logic/MATLAB Function1 ==
  data: tracks input; relativeDistance output; lane input; egoInfo input; distanceToIntersection input; relativeVelocity output; mioTrackIndex output; maxDistance parameter; posSelector parameter; velSelector parameter; crossOverVehicleAlert output
function [relativeDistance,relativeVelocity,mioTrackIndex, crossOverVehicleAlert] = helperFindMIO(tracks, lane, egoInfo, distanceToIntersection,maxDistance, posSelector, velSelector)
    % helperFindMIO Find's the most Important object and compute the
    % relative distance and relative velocity. The MIO can be lead car or
    % it can be a crossover vehicle

    % NOTE: This is a helper function for example purposes and may be removed or
    % modified in the future.

    % Copyright 2021 The MathWorks, Inc.

    % Initialize outputs and parameters
    relativeDistance = Inf;
    relativeVelocity = Inf;
    mioTrackIndex    = -1;
    crossOverVehicleAlert = false;

    % Initialise track related Information
    coder.varsize('confirmedTracks');
    coder.varsize('posTrack');
    coder.varsize('velTrack');
    confirmedTracks = tracks.Tracks(1);
    posTrack = [0 0];
    velTrack = [0 0];

    % get track position and velocity
    if tracks.NumTracks>0
        confirmedTracks = tracks.Tracks(1:tracks.NumTracks);
        posTrack = getTrackPositions(confirmedTracks,posSelector);
        velTrack = getTrackVelocities(confirmedTracks,velSelector);
    end

    % Initialize MIO Index
    mioIndex    = 0;
    crossOverMIOIndex = 0;

    % Initialize Position for lead and crossover vehicle
    mioPos = inf;
    mioCrossPos = inf;

    % Initialize threshold for relative distance
    minDist        = maxDistance;
    minCrossDist   = maxDistance;
    % Initialize minimum distance to intersection
    minDistToInter = 60; % meters
    % Initialize minimum time gap
    minTgap = 5;

    % Initialize Velocity for lead and crossover vehicle
    mioVel = inf;
    mioCrossVel = inf;

    % Time for path prediction
    tpp = 20;

    % If lane detection is not available, the ego car is assumed to be located
    % in the middle of its lane. The lane width is assumed to be 3.6m, typical
    % highway lane width.
    
    % Lane Info
    laneWidth = 3.6;
    halfLaneWidth = laneWidth/2;
    
    % Compute the left and right lane boundaries
    if lane.Left.Strength > 0.01
        lb = [lane.Left.CurvatureDerivative/6,...
            lane.Left.Curvature/2,...
            lane.Left.HeadingAngle,...
            lane.Left.LateralOffset];
    else
        lb = single([0,0,0,halfLaneWidth]);
    end
    
    if lane.Right.Strength > 0.01
        rb = [lane.Right.CurvatureDerivative/6,...
            lane.Right.Curvature/2,...
            lane.Right.HeadingAngle,...
            lane.Right.LateralOffset];
    else
        rb = single([0,0,0,-halfLaneWidth]);
    end

    
    for i = 1:tracks.NumTracks    
        targetPos = posTrack(i,:);
        targetVel = velTrack(i,:);

        egoPos = [egoInfo.Position(1:2)];
        egoYaw = egoInfo.Yaw;
        egoVelocity = egoInfo.Velocity;
        rotmat = [cosd(egoYaw), -sind(egoYaw); sind(egoYaw), cosd(egoYaw)];
        
        locations = (targetPos - egoPos)*rotmat;
        relativeDistance = locations(1); % Longitudinal position
        latPos = locations(2);           % Lateral position

        % Check Of MIO infront of ego
        if relativeDistance < minDist && relativeDistance > 0 % No point checking otherwise
            latLeftLane  = polyval(lb,relativeDistance); % lateral position of left lane
            latRightLane = polyval(rb,relativeDistance); % lateral position of right lane            
            % Find a new MIO track
            if (latRightLane <= latPos) && (latPos <= latLeftLane)
                minDist  = relativeDistance;
                mioIndex = double(confirmedTracks(i).TrackID);
                mioPos   = relativeDistance;
                mioVel   = double(norm(targetVel))-double(norm([egoVelocity(1),egoVelocity(2)]));
            end
        end
        % Check for crossover MIO vehicle when distance to intersection is 
        % less than threshold 
        if distanceToIntersection>0 && distanceToIntersection<minDistToInter
            % Compute target heading 
            targetHeading = rad2deg(cart2pol(targetVel(2),targetVel(1)));
            targetHeading = rem(targetHeading+360,360);
            % Compute ego heading
            egoHeading    = rem((450-rem(360+egoYaw,360)),360);
            % Check if the vehicle approaches from left or right, excluding
            % the forward and rear vehicles
            leftFlag  = (isAngleBetween(targetHeading,rem(egoHeading+40,360),rem(egoHeading+140,360))) && (latPos>=0);
            rightFlag = (isAngleBetween(targetHeading,rem(egoHeading+220,360),rem(egoHeading+320,360))) && (latPos<0);

            if leftFlag || rightFlag
                % Estimate target path
                targetSpeed   = norm(targetVel);
                targetPath    = vehiclePath(tpp,targetHeading,targetSpeed,[targetPos(1),targetPos(2)]);
                
                % Estimate ego path
                egoSpeed      = double(norm([egoVelocity(1),egoVelocity(2)]));
                if egoSpeed < 1.5
                    egoSpeed = 9;
                end
                egoPath       = vehiclePath(tpp,egoHeading,egoSpeed,[egoPos(1),egoPos(2)]);

                % Check for intersection between ego and target path
                intersection = intersectionPoint(targetPath,egoPath);

                % If intersection exist get the distance and velocity
                if ~isempty(intersection)
                    targetDist = norm(targetPath(1,:) - intersection);
                    egoDist    = norm(egoPath(1,:) - intersection);
                    targetTime = targetDist/targetSpeed;
                    egoTime    = egoDist/egoSpeed;
                    % If ego and target vehicle reach the intersection
                    % point within the minimum time gap and the ego
                    % distance to intersection is less than minimum
                    % crossover distance, consider it to be an MIO and
                    % compute the relative distance and velocity.

                    % For Cross Over Vehicle Condition,
                    % The relative distance is considered to be the
                    % distance between ego to intersection point and the
                    % relative velocity is considered to be the ego's
                    % velocity towards the intersection point.
                    if (abs(egoTime-targetTime)<=minTgap) && egoDist<minCrossDist
                        minCrossDist = egoDist;
                        mioCrossPos  = min(egoDist,distanceToIntersection);
                        mioCrossVel  = -1*double(norm([egoVelocity(1),egoVelocity(2)]));
                        crossOverMIOIndex = double(confirmedTracks(i).TrackID);
                    end
                end
            end
            
        end
    end
    if mioIndex > 0 || crossOverMIOIndex>0
        % Output:If MIO is lead vehicle
        if mioPos < mioCrossPos
            % Longitudinal position of the lead car
            relativeDistance = mioPos;
            % Longitudinal velocity of the lead car
            relativeVelocity = mioVel;
            mioTrackIndex = mioIndex;
        % Output:If MIO is crossover vehicle
        else
            % Distance to intersection point
            relativeDistance = mioCrossPos;
            % Ego velocity towards the intersection point
            relativeVelocity = mioCrossVel;
            mioTrackIndex    = crossOverMIOIndex;
            crossOverVehicleAlert = true;
        end
    else
        % Output: If no MIO
        relativeDistance = inf; 
        relativeVelocity = inf; 
        mioTrackIndex    = -1;
    end
end

% Estimate the vehicle's path based on heading, speed and current position
function path = vehiclePath(tpp,heading,speed,initialPos)
    distTravelled  = speed*tpp;
    xOffset = distTravelled*sind(double(heading));
    yOffset = distTravelled*cosd(double(heading));
    path    = double([initialPos(1) initialPos(2);initialPos(1)+xOffset initialPos(2)+yOffset]);
end

% Compute the Intersection Point between two paths
function intersection = intersectionPoint(targetPath,egoPath)
    intersection = zeros(0,2);
    x1 = double([targetPath(1,1),targetPath(2,1)]);
    y1 = double([targetPath(1,2),targetPath(2,2)]);
    x2 = double([egoPath(1,1),egoPath(2,1)]);
    y2 = double([egoPath(1,2),egoPath(2,2)]);
    
    A = [x1(2)-x1(1)       0       -1   0;      
              0       x2(2)-x2(1)  -1   0;   
         y1(2)-y1(1)       0        0  -1;      
              0       y2(2)-y2(1)   0  -1];      
          
    B = [-x1(1);
         -x2(1);
         -y1(1);
         -y2(1)];
    % Compute solution only if matrix is not singular
    if rank(A)==size(A,2)
        T = (eye(4)/A)*B;
        if ((0<=T(1)) && (T(1)<1)) && ((0<=T(2)) && (T(2)<1))
            intersection = [T(3),T(4)];
        end
    end
end

% Check if an anlge lies between lower bound and upper bound
function flag = isAngleBetween(angle,lb,ub)
    flag=(lb<=angle & angle<=ub)|(((0<=angle & angle<=ub)|lb <= angle) & lb>ub);
end
